simulink model "ImuCalibrator3Pass"  (R2018a)
settings: Solver=FixedStepDiscrete  StartTime=0.0  StopTime=inf  FixedStep=1/Fss  RelTol=1e-3
PreLoadFcn:
  | busDef
  | Fss = 1125;
  | Fss = 2100;
InitFcn:
  | modelDef = getModelDef(true);
undefined symbols (not defined in the file or in its folder): df, dw, Ggyr, Macc, Mgyr, numStates
libraries: simulink x15, vrlib x15, dspsigops x6, dspindex x6, dspinverses x6, dspstat3 x3, simulink_extras x3, dspmtrx3 x3, dspsrcs4 x3, dspmathops x3, dspswit3 x1
(part 1 of 4)
settings Model: Creator=Eric  LastModifiedBy=efoxlin
settings OptimizationCC: DefaultParameterBehavior=Inlined  InlineInvariantSignals=on  PassReuseOutputArgsAs=Individual arguments
settings DebuggingCC: ParameterTunabilityLossMsg=error  UnconnectedOutputMsg=none
settings SFSimCC: MATLABDynamicMemAlloc=off
settings RTWCC: SystemTargetFile=ert.tlc  TemplateMakefile=ert_default_tmf  GenerateReport=on  Toolchain=Microsoft Visual C++ 2017 v15.0 | nmake (64-bit Windows)  BuildConfiguration=Faster Runs  IncludeHyperlinkInReport=on  LaunchReport=on  GenerateTraceInfo=on  GenerateTraceReport=on  GenerateTraceReportSl=on  GenerateTraceReportSf=on  GenerateTraceReportEml=on
settings CodeAppCC: ForceParamTrailComments=on  IgnoreCustomStorageClasses=off  OperatorAnnotations=on  SimulinkDataObjDesc=on  SFDataObjDesc=on  InsertBlockDesc=on
settings ERTTargetCC: TargetLangStandard=C99 (ISO)  GenerateSampleERTMain=on  SupportComplex=off  SupportNonInlinedSFcns=on  SupportVariableSizeSignals=on  InlinedParameterPlacement=NonHierarchical  ERTCustomFileTemplate=example_file_process.tlc

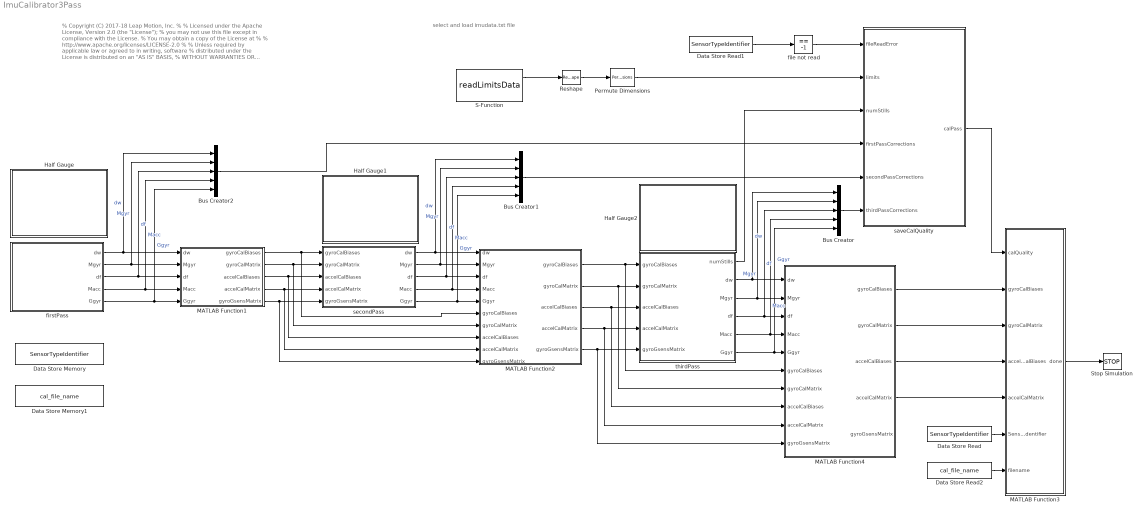
== system ImuCalibrator3Pass ==
  note: select and load imudata.txt file
  note: % Copyright (C) 2017-18 Leap Motion, Inc.
      | %
      | %    Licensed under the Apache License, Version 2.0 (the "License");
      | %    you may not use this file except in compliance with the License.
      | %    You may obtain a copy of the License at
      | %
      | %        http://www.apache.org/licenses/LICENSE-2.0
      | %
      | %    Unless required by applicable law or agreed to in writing, software
      | %    distributed under the License is distributed on an "AS IS" BASIS,
      | %    WITHOUT WARRANTIES OR CONDITIONS OF ANY KIND, either express or implied.
      | %    See the License for the specific language governing permissions and
      | %    limitations under the License.
      | % Author: Eric Foxlin
  Bus Creator : BusCreator  Inputs=dw,Mgyr,df,Macc,Ggyr
  Bus Creator1 : BusCreator  Inputs=dw,Mgyr,df,Macc,Ggyr
  Bus Creator2 : BusCreator  Inputs=dw,Mgyr,df,Macc,Ggyr
  Data Store Memory : DataStoreMemory  DataStoreName=SensorTypeIdentifier  ReadBeforeWriteMsg=warning  WriteAfterWriteMsg=warning  WriteAfterReadMsg=warning  InitialValue=-1  ShowAdditionalParam=off  OutDataTypeStr=int32
  Data Store Memory1 : DataStoreMemory  DataStoreName=cal_file_name  ReadBeforeWriteMsg=warning  WriteAfterWriteMsg=warning  WriteAfterReadMsg=warning  InitialValue=[76,69,48,48,48,48,48,48,48,48,48,48,48,48,48,48,48,48,45,48,48,48,48,45,48,48,48,48,48,48,48,48,48,48,45,105,109,117,46,106,115,111,110]  ShowAdditionalParam=off  OutDataTypeStr=uint8  Dimensions=[1,43]
  Data Store Read : DataStoreRead  Priority=7  DataStoreName=SensorTypeIdentifier
  Data Store Read1 : DataStoreRead  Priority=7  DataStoreName=SensorTypeIdentifier
  Data Store Read2 : DataStoreRead  Priority=7  DataStoreName=cal_file_name
  Half Gauge : Subsystem  DialogController=hmiCreateDDGDialog  IsWebBlock=on  mask(MWDashboardBlock){webBlockId=50db2cba-56c0-46f6-8461-fb1f4f79e19a, webBlockType=semicirculargauge, ShowInLibBrowser=on, ShowInitialText=on, HMISrcModelName=ImuCalibrator3Pass}
      mask prompts: webBlockId "WebBlock Id"; webBlockType "WebBlock Type"; HMISrcModelName "Source Model"
      mask help: SimulinkHMI:dialogs:SemicircularGaugeDialogDesc
      mask Help: helpview([docroot '/mapfiles/simulink.map'], 'hmi_half_gauge')
      mask Display:
      | if strcmp(get_param(bdroot(gcb),'BlockDiagramType'), 'library')
      |     image([(matlabroot) '/toolbox/simulink/hmi/icons/SemicircularGauge.png']);
      | end
  Half Gauge1 : Subsystem  DialogController=hmiCreateDDGDialog  IsWebBlock=on  mask(MWDashboardBlock){webBlockId=ea91a535-1150-4075-a79a-66e57a6dcc36, webBlockType=semicirculargauge, ShowInLibBrowser=on, ShowInitialText=on, HMISrcModelName=ImuCalibrator3Pass}
      mask prompts: webBlockId "WebBlock Id"; webBlockType "WebBlock Type"; HMISrcModelName "Source Model"
      mask help: SimulinkHMI:dialogs:SemicircularGaugeDialogDesc
      mask Help: helpview([docroot '/mapfiles/simulink.map'], 'hmi_half_gauge')
      mask Display:
      | if strcmp(get_param(bdroot(gcb),'BlockDiagramType'), 'library')
      |     image([(matlabroot) '/toolbox/simulink/hmi/icons/SemicircularGauge.png']);
      | end
  Half Gauge2 : Subsystem  DialogController=hmiCreateDDGDialog  IsWebBlock=on  mask(MWDashboardBlock){webBlockId=9f86d34f-810e-44c4-a7af-c4dea1104fb5, webBlockType=semicirculargauge, ShowInLibBrowser=on, ShowInitialText=on, HMISrcModelName=ImuCalibrator3Pass}
      mask prompts: webBlockId "WebBlock Id"; webBlockType "WebBlock Type"; HMISrcModelName "Source Model"
      mask help: SimulinkHMI:dialogs:SemicircularGaugeDialogDesc
      mask Help: helpview([docroot '/mapfiles/simulink.map'], 'hmi_half_gauge')
      mask Display:
      | if strcmp(get_param(bdroot(gcb),'BlockDiagramType'), 'library')
      |     image([(matlabroot) '/toolbox/simulink/hmi/icons/SemicircularGauge.png']);
      | end
  MATLAB Function1 : MATLAB Function  TreatAsAtomicUnit=on
  MATLAB Function2 : MATLAB Function  TreatAsAtomicUnit=on
  MATLAB Function3 : MATLAB Function  TreatAsAtomicUnit=on
  MATLAB Function4 : MATLAB Function  TreatAsAtomicUnit=on
  Permute Dimensions : PermuteDimensions
  Reshape : Reshape  OutputDimensionality=Customize  OutputDimensions=[6,3]
  S-Function : S-Function  FunctionName=readLimitsData  Parameters=-1  SFunctionDeploymentMode=off  EnableBusSupport=off
  Stop Simulation : Stop
  file not read : simulink/Logic and Bit Operations/Compare To Constant  relop===  const=-1  OutDataTypeStr=boolean
  firstPass : Subsystem  Priority=1
      mask init:
      | imuPar = getImuPar('lmvpUncalibrated');
  saveCalQuality : MATLAB Function  TreatAsAtomicUnit=on
  secondPass : Subsystem
      mask init:
      | imuPar = getImuPar('lmvp2ndPassCalibration');
  thirdPass : Subsystem
      mask init:
      | imuPar = getImuPar('lmvp2ndPassCalibration');
  wires:
  MATLAB Function1/1(gyroCalBiases) -> MATLAB Function2/6("gyroCalBiases "), secondPass/1(gyroCalBiases)
  MATLAB Function1/2(gyroCalMatrix) -> MATLAB Function2/7("gyroCalMatrix "), secondPass/2(gyroCalMatrix)
  MATLAB Function1/5(gyroGsensMatrix) -> MATLAB Function2/10("gyroGsensMatrix "), secondPass/5(gyroGsensMatrix)
  MATLAB Function1/3(accelCalBiases) -> MATLAB Function2/8("accelCalBiases "), secondPass/3(accelCalBiases)
  MATLAB Function1/4(accelCalMatrix) -> MATLAB Function2/9("accelCalMatrix "), secondPass/4(accelCalMatrix)
  MATLAB Function2/1(gyroCalBiases) -> MATLAB Function4/6("gyroCalBiases "), thirdPass/1(gyroCalBiases)
  MATLAB Function2/2(gyroCalMatrix) -> MATLAB Function4/7("gyroCalMatrix "), thirdPass/2(gyroCalMatrix)
  MATLAB Function2/3(accelCalBiases) -> MATLAB Function4/8("accelCalBiases "), thirdPass/3(accelCalBiases)
  MATLAB Function2/4(accelCalMatrix) -> MATLAB Function4/9("accelCalMatrix "), thirdPass/4(accelCalMatrix)
  MATLAB Function2/5(gyroGsensMatrix) -> MATLAB Function4/10("gyroGsensMatrix "), thirdPass/5(gyroGsensMatrix)
  thirdPass/2(dw) -> Bus Creator/1, MATLAB Function4/1(dw)  "dw"
  thirdPass/3(Mgyr) -> Bus Creator/2, MATLAB Function4/2(Mgyr)  "Mgyr"
  thirdPass/4(df) -> Bus Creator/3, MATLAB Function4/3(df)  "df"
  thirdPass/5(Macc) -> Bus Creator/4, MATLAB Function4/4(Macc)  "Macc"
  MATLAB Function4/1(gyroCalBiases) -> MATLAB Function3/2(gyroCalBiases)
  thirdPass/6(Ggyr) -> Bus Creator/5, MATLAB Function4/5(Ggyr)  "Ggyr"
  MATLAB Function3/1(done) -> Stop Simulation/1
  Bus Creator/1 -> saveCalQuality/6(thirdPassCorrections)
  MATLAB Function4/2(gyroCalMatrix) -> MATLAB Function3/3(gyroCalMatrix)
  MATLAB Function4/3(accelCalBiases) -> MATLAB Function3/4(accelCalBiases)
  MATLAB Function4/4(accelCalMatrix) -> MATLAB Function3/5(accelCalMatrix)
  saveCalQuality/1(calPass) -> MATLAB Function3/1(calQuality)
  secondPass/5(Ggyr) -> Bus Creator1/5, MATLAB Function2/5(Ggyr)  "Ggyr"
  secondPass/3(df) -> Bus Creator1/3, MATLAB Function2/3(df)  "df"
  secondPass/4(Macc) -> Bus Creator1/4, MATLAB Function2/4(Macc)  "Macc"
  secondPass/2(Mgyr) -> Bus Creator1/2, MATLAB Function2/2(Mgyr)  "Mgyr"
  secondPass/1(dw) -> Bus Creator1/1, MATLAB Function2/1(dw)  "dw"
  firstPass/1(dw) -> Bus Creator2/1, MATLAB Function1/1(dw)  "dw"
  firstPass/2(Mgyr) -> Bus Creator2/2, MATLAB Function1/2(Mgyr)  "Mgyr"
  firstPass/4(Macc) -> Bus Creator2/4, MATLAB Function1/4(Macc)  "Macc"
  firstPass/3(df) -> Bus Creator2/3, MATLAB Function1/3(df)  "df"
  firstPass/5(Ggyr) -> Bus Creator2/5, MATLAB Function1/5(Ggyr)  "Ggyr"
  Bus Creator1/1 -> saveCalQuality/5(secondPassCorrections)
  Bus Creator2/1 -> saveCalQuality/4(firstPassCorrections)
  Data Store Read/1 -> MATLAB Function3/6(SensorTypeIdentifier)
  Data Store Read1/1 -> file not read/1
  file not read/1 -> saveCalQuality/1(fileReadError)
  thirdPass/1(numStills) -> saveCalQuality/3(numStills)
  Permute Dimensions/1 -> saveCalQuality/2(limits)
  S-Function/1 -> Reshape/1
  Reshape/1 -> Permute Dimensions/1
  Data Store Read2/1 -> MATLAB Function3/7(filename)

== system ImuCalibrator3Pass/Half Gauge ==

== system ImuCalibrator3Pass/Half Gauge1 ==

== system ImuCalibrator3Pass/Half Gauge2 ==

== system ImuCalibrator3Pass/firstPass ==
  AINS : Subsystem  TreatAsAtomicUnit=on
  Binary File Reader : dspsrcs4/Binary File Reader  Commented=on  Filename=GyroAccelDtFloat32.bin  HeaderStructure=struct([])  DataType=single  SamplesPerFrame=1  IsDataComplex=off  NumChannels=7  OutputEOF=on  SampleTime=-1  SimulateUsing=Code generation
      settings: SourceProductName=DSP System Toolbox  SourceProductBaseCode=DS
  Bus Selector : BusSelector  OutputSignals=dw,Mgyr,df,Macc,Ggyr
  Compare To Zero : simulink/Logic and Bit Operations/Compare To Zero  relop===  OutDataTypeStr=boolean
  Constant : Constant  Value=int32(4096)
  Cumulative time : dspmathops/Cumulative Sum  dim=Channels (running sum)  reset_popup=None  roundingMode=Floor  overflowMode=off  outputDataTypeStr=Inherit: Same as accumulator  outputMin=[]  outputMax=[]  outputLastDataTypeStr=Inherit: Same as accumulator
      settings: SourceProductName=DSP System Toolbox
  Data Type Conversion : DataTypeConversion
  Demux : Demux  Outputs=[3 3 1]
  Dt : Selector  InputPortWidth=7  IndexOptions=Index vector (dialog)  Indices=7  OutputSizes=1
  Logical Operator : Logic  Operator=NOT  AllPortsSameDT=off  OutDataTypeStr=boolean
  MATLAB Function1 : MATLAB Function  Commented=on  TreatAsAtomicUnit=on
  Math Function : Math  Operator=mod  SaturateOnIntegerOverflow=on
  Reshape : Reshape  OutputDimensionality=Column vector (2-D)
  Scope1 : Scope
  Scope10 : Scope
  Scope3 : Scope
  To Workspace : ToWorkspace  Commented=on  VariableName=simout  SaveFormat=Timeseries  SampleTime=-1
      settings: Save2DSignal=2-D array (concatenate along first dimension)
  While Iterator : WhileIterator  MaxIters=500000  WhileBlockType=do-while  ShowIterationPort=on
  printTime : Subsystem
  readImuData : Subsystem
  dw : Outport
  Mgyr : Outport  Port=2
  df : Outport  Port=3
  Macc : Outport  Port=4
  Ggyr : Outport  Port=5
  wires:
  AINS/1(filterOut) -> Bus Selector/1, To Workspace/1  "filterOut"
  Demux/1 -> AINS/1(w_ib^b), Scope1/1
  Demux/3 -> Scope3/1, AINS/3(Dt)
  Demux/2 -> AINS/2(f_ib^b), Scope10/1
  Bus Selector/1 -> dw/1  "<dw>"
  Bus Selector/2 -> Mgyr/1  "<Mgyr>"
  Bus Selector/3 -> df/1  "<df>"
  Bus Selector/4 -> Macc/1  "<Macc>"
  Bus Selector/5 -> Ggyr/1  "<Ggyr>"
  While Iterator/1 -> Math Function/1
  Math Function/1 -> Compare To Zero/1
  Constant/1 -> Math Function/2
  Cumulative time/1 -> printTime/1(time)  "firstPassTime"
  readImuData/1(GyrosAccelsDt) -> Data Type Conversion/1
  Reshape/1 -> Demux/1
  readImuData/2(EOF) -> Logical Operator/1
  Logical Operator/1 -> While Iterator/1
  Data Type Conversion/1 -> Dt/1, Reshape/1
  Compare To Zero/1 -> printTime/Enable
  Dt/1 -> Cumulative time/1

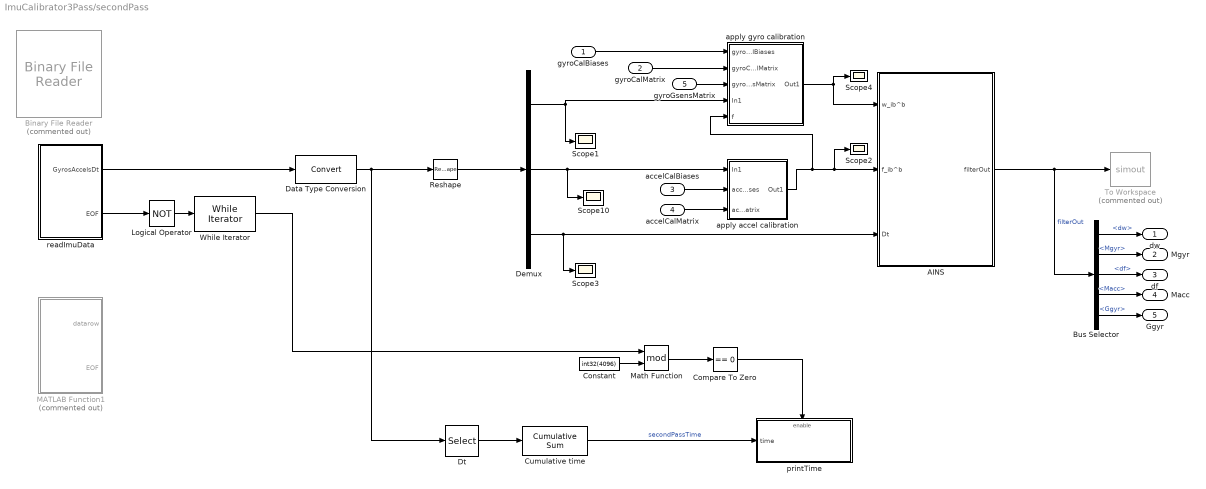
== system ImuCalibrator3Pass/secondPass ==
  gyroCalBiases : Inport
  gyroCalMatrix : Inport  Port=2
  accelCalBiases : Inport  Port=3
  accelCalMatrix : Inport  Port=4
  gyroGsensMatrix : Inport  Port=5
  AINS : Subsystem  TreatAsAtomicUnit=on
  Binary File Reader : dspsrcs4/Binary File Reader  Commented=on  Filename=GyroAccelDtFloat32.bin  HeaderStructure=struct([])  DataType=single  SamplesPerFrame=1  IsDataComplex=off  NumChannels=7  OutputEOF=on  SampleTime=-1  SimulateUsing=Code generation
      settings: SourceProductName=DSP System Toolbox  SourceProductBaseCode=DS
  Bus Selector : BusSelector  OutputSignals=dw,Mgyr,df,Macc,Ggyr
  Compare To Zero : simulink/Logic and Bit Operations/Compare To Zero  relop===  OutDataTypeStr=boolean
  Constant : Constant  Value=int32(4096)
  Cumulative time : dspmathops/Cumulative Sum  dim=Channels (running sum)  reset_popup=None  roundingMode=Floor  overflowMode=off  outputDataTypeStr=Inherit: Same as accumulator  outputMin=[]  outputMax=[]  outputLastDataTypeStr=Inherit: Same as accumulator
      settings: SourceProductName=DSP System Toolbox
  Data Type Conversion : DataTypeConversion
  Demux : Demux  Outputs=[3 3 1]
  Dt : Selector  InputPortWidth=7  IndexOptions=Index vector (dialog)  Indices=7  OutputSizes=1
  Logical Operator : Logic  Operator=NOT  AllPortsSameDT=off  OutDataTypeStr=boolean
  MATLAB Function1 : MATLAB Function  Commented=on  TreatAsAtomicUnit=on
  Math Function : Math  Operator=mod  SaturateOnIntegerOverflow=on
  Reshape : Reshape  OutputDimensionality=Column vector (2-D)
  Scope{1..4,10} (5 alike) : Scope
  To Workspace : ToWorkspace  Commented=on  VariableName=simout  SaveFormat=Timeseries  SampleTime=-1
      settings: Save2DSignal=2-D array (concatenate along first dimension)
  While Iterator : WhileIterator  MaxIters=500000  WhileBlockType=do-while  ShowIterationPort=on
  apply accel calibration : Subsystem  TreatAsAtomicUnit=on
  apply gyro calibration : Subsystem  TreatAsAtomicUnit=on
  printTime : Subsystem
  readImuData : Subsystem
  dw : Outport
  Mgyr : Outport  Port=2
  df : Outport  Port=3
  Macc : Outport  Port=4
  Ggyr : Outport  Port=5
  wires:
  Compare To Zero/1 -> printTime/Enable
  Data Type Conversion/1 -> Dt/1, Reshape/1
  Logical Operator/1 -> While Iterator/1
  readImuData/2(EOF) -> Logical Operator/1
  Reshape/1 -> Demux/1
  readImuData/1(GyrosAccelsDt) -> Data Type Conversion/1
  Cumulative time/1 -> printTime/1(time)  "secondPassTime"
  Constant/1 -> Math Function/2
  Math Function/1 -> Compare To Zero/1
  While Iterator/1 -> Math Function/1
  Bus Selector/5 -> Ggyr/1  "<Ggyr>"
  Bus Selector/4 -> Macc/1  "<Macc>"
  Bus Selector/3 -> df/1  "<df>"
  Bus Selector/2 -> Mgyr/1  "<Mgyr>"
  Bus Selector/1 -> dw/1  "<dw>"
  apply accel calibration/1(Out1) -> apply gyro calibration/5(f), Scope2/1, AINS/2(f_ib^b)
  Demux/3 -> AINS/3(Dt), Scope3/1
  apply gyro calibration/1(Out1) -> AINS/1(w_ib^b), Scope4/1
  Demux/1 -> apply gyro calibration/4(In1), Scope1/1
  Demux/2 -> apply accel calibration/1(In1), Scope10/1
  AINS/1(filterOut) -> To Workspace/1, Bus Selector/1  "filterOut"
  gyroCalBiases/1 -> apply gyro calibration/1(gyroCalBiases)
  gyroCalMatrix/1 -> apply gyro calibration/2(gyroCalMatrix)
  gyroGsensMatrix/1 -> apply gyro calibration/3(gyroGsensMatrix)
  accelCalBiases/1 -> apply accel calibration/2(accelCalBiases)
  accelCalMatrix/1 -> apply accel calibration/3(accelCalMatrix)
  Dt/1 -> Cumulative time/1

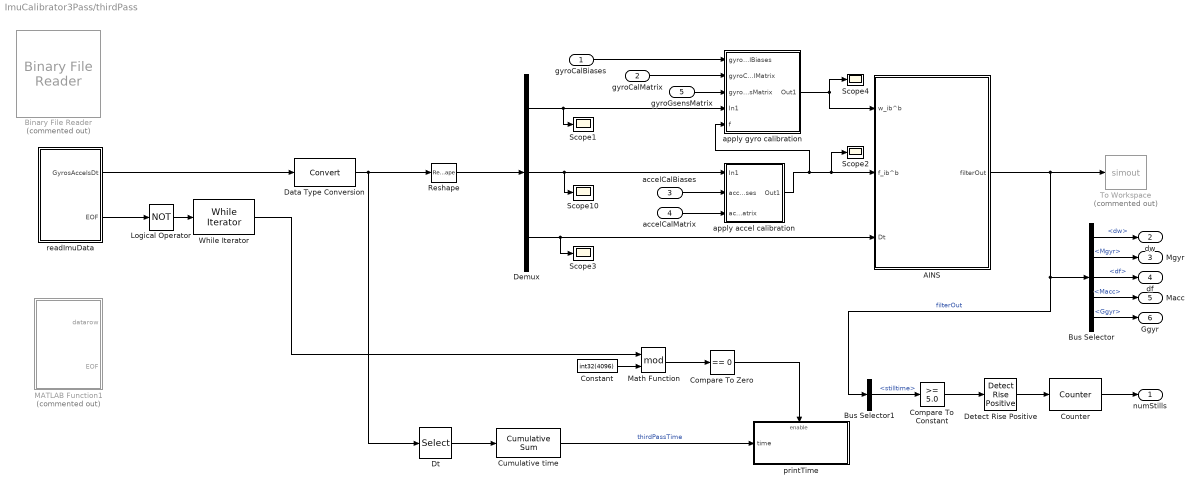
== system ImuCalibrator3Pass/thirdPass ==
  gyroCalBiases : Inport
  gyroCalMatrix : Inport  Port=2
  accelCalBiases : Inport  Port=3
  accelCalMatrix : Inport  Port=4
  gyroGsensMatrix : Inport  Port=5
  AINS : Subsystem  TreatAsAtomicUnit=on
  Binary File Reader : dspsrcs4/Binary File Reader  Commented=on  Filename=GyroAccelDtFloat32.bin  HeaderStructure=struct([])  DataType=single  SamplesPerFrame=1  IsDataComplex=off  NumChannels=7  OutputEOF=on  SampleTime=-1  SimulateUsing=Code generation
      settings: SourceProductName=DSP System Toolbox  SourceProductBaseCode=DS
  Bus Selector : BusSelector  OutputSignals=dw,Mgyr,df,Macc,Ggyr
  Bus Selector1 : BusSelector  OutputSignals=stilltime
  Compare To Constant : simulink/Logic and Bit Operations/Compare To Constant  relop=>=  const=5.0  OutDataTypeStr=boolean
  Compare To Zero : simulink/Logic and Bit Operations/Compare To Zero  relop===  OutDataTypeStr=boolean
  Constant : Constant  Value=int32(4096)
  Counter : dspswit3/Counter  Direction=Up  CountEvent=Non-zero sample  CounterSize=User defined  MaxCount=255  InitialCount=0  Output=Count  HitValue=32  ResetInput=off  SamplesPerFrame=1  Ts=1  CntDtype=double  HitDtype=Logical
  Cumulative time : dspmathops/Cumulative Sum  dim=Channels (running sum)  reset_popup=None  roundingMode=Floor  overflowMode=off  outputDataTypeStr=Inherit: Same as accumulator  outputMin=[]  outputMax=[]  outputLastDataTypeStr=Inherit: Same as accumulator
      settings: SourceProductName=DSP System Toolbox
  Data Type Conversion : DataTypeConversion
  Demux : Demux  Outputs=[3 3 1]
  Detect Rise Positive : simulink/Logic and Bit Operations/Detect Rise Positive  vinit=0  OutDataTypeStr=boolean
  Dt : Selector  InputPortWidth=7  IndexOptions=Index vector (dialog)  Indices=7  OutputSizes=1
  Logical Operator : Logic  Operator=NOT  AllPortsSameDT=off  OutDataTypeStr=boolean
  MATLAB Function1 : MATLAB Function  Commented=on  TreatAsAtomicUnit=on
  Math Function : Math  Operator=mod  SaturateOnIntegerOverflow=on
  Reshape : Reshape  OutputDimensionality=Column vector (2-D)
  Scope{1..4,10} (5 alike) : Scope
  To Workspace : ToWorkspace  Commented=on  VariableName=simout  SaveFormat=Timeseries  SampleTime=-1
      settings: Save2DSignal=2-D array (concatenate along first dimension)
  While Iterator : WhileIterator  MaxIters=500000  WhileBlockType=do-while  ShowIterationPort=on
  apply accel calibration : Subsystem  TreatAsAtomicUnit=on
  apply gyro calibration : Subsystem  TreatAsAtomicUnit=on
  printTime : Subsystem
  readImuData : Subsystem
  numStills : Outport  InitialOutput=0
  dw : Outport  Port=2
  Mgyr : Outport  Port=3
  df : Outport  Port=4
  Macc : Outport  Port=5
  Ggyr : Outport  Port=6
  wires:
  accelCalMatrix/1 -> apply accel calibration/3(accelCalMatrix)
  accelCalBiases/1 -> apply accel calibration/2(accelCalBiases)
  gyroGsensMatrix/1 -> apply gyro calibration/3(gyroGsensMatrix)
  gyroCalMatrix/1 -> apply gyro calibration/2(gyroCalMatrix)
  gyroCalBiases/1 -> apply gyro calibration/1(gyroCalBiases)
  AINS/1(filterOut) -> Bus Selector1/1, Bus Selector/1, To Workspace/1  "filterOut"
  Demux/2 -> Scope10/1, apply accel calibration/1(In1)
  Demux/1 -> Scope1/1, apply gyro calibration/4(In1)
  apply gyro calibration/1(Out1) -> Scope4/1, AINS/1(w_ib^b)
  Demux/3 -> Scope3/1, AINS/3(Dt)
  apply accel calibration/1(Out1) -> AINS/2(f_ib^b), Scope2/1, apply gyro calibration/5(f)
  Bus Selector/1 -> dw/1  "<dw>"
  Bus Selector/2 -> Mgyr/1  "<Mgyr>"
  Bus Selector/3 -> df/1  "<df>"
  Bus Selector/4 -> Macc/1  "<Macc>"
  Bus Selector/5 -> Ggyr/1  "<Ggyr>"
  While Iterator/1 -> Math Function/1
  Math Function/1 -> Compare To Zero/1
  Constant/1 -> Math Function/2
  Cumulative time/1 -> printTime/1(time)  "thirdPassTime"
  readImuData/1(GyrosAccelsDt) -> Data Type Conversion/1
  Reshape/1 -> Demux/1
  readImuData/2(EOF) -> Logical Operator/1
  Logical Operator/1 -> While Iterator/1
  Data Type Conversion/1 -> Dt/1, Reshape/1
  Compare To Zero/1 -> printTime/Enable
  Dt/1 -> Cumulative time/1
  Bus Selector1/1 -> Compare To Constant/1  "<stilltime>"
  Compare To Constant/1 -> Detect Rise Positive/1
  Detect Rise Positive/1 -> Counter/1
  Counter/1 -> numStills/1

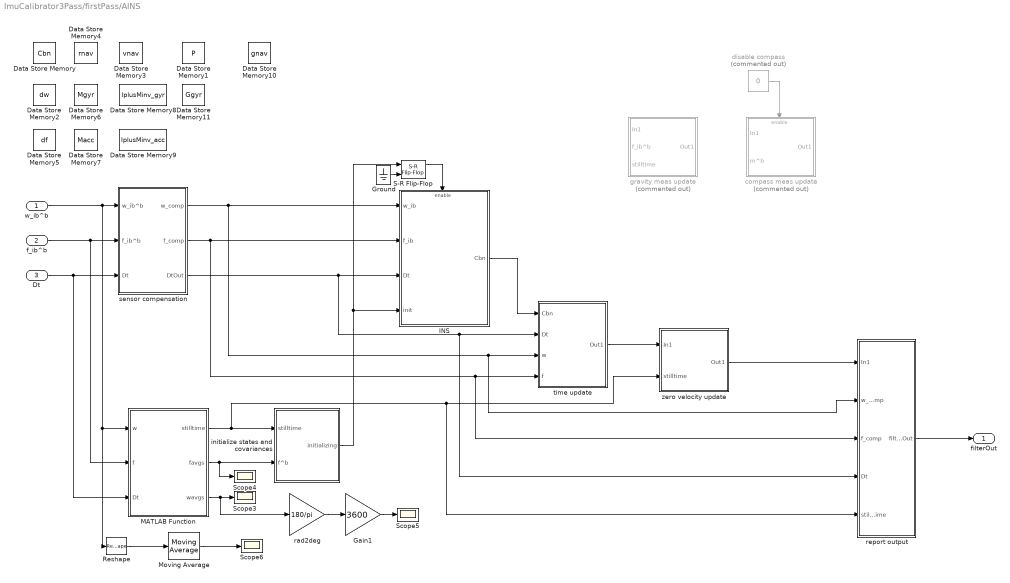
== system ImuCalibrator3Pass/firstPass/AINS ==
  w_ib^b : Inport  Unit=rad/s
  f_ib^b : Inport  Port=2  Unit=m/s^2  PortDimensions=3
  Dt : Inport  Port=3  Unit=rad/s
  Data Store Memory : DataStoreMemory  DataStoreName=Cbn  ReadBeforeWriteMsg=warning  WriteAfterWriteMsg=warning  WriteAfterReadMsg=warning  InitialValue=eye(3)  VectorParams1D=off  ShowAdditionalParam=off
  Data Store Memory1 : DataStoreMemory  DataStoreName=P  ReadBeforeWriteMsg=warning  WriteAfterWriteMsg=warning  WriteAfterReadMsg=warning  InitialValue=eye(modelDef.numStates)*1e-12  ShowAdditionalParam=off
  Data Store Memory10 : DataStoreMemory  DataStoreName=gnav  ReadBeforeWriteMsg=warning  WriteAfterWriteMsg=warning  WriteAfterReadMsg=warning  InitialValue=[0;0; 9.8065]  VectorParams1D=off  ShowAdditionalParam=off
  Data Store Memory11 : DataStoreMemory  DataStoreName=Ggyr  ReadBeforeWriteMsg=warning  WriteAfterWriteMsg=warning  WriteAfterReadMsg=warning  InitialValue=zeros(3,3)  VectorParams1D=off  ShowAdditionalParam=off
  Data Store Memory2 : DataStoreMemory  DataStoreName=dw  ReadBeforeWriteMsg=warning  WriteAfterWriteMsg=warning  WriteAfterReadMsg=warning  InitialValue=[0;0;0]  VectorParams1D=off  ShowAdditionalParam=off
  Data Store Memory3 : DataStoreMemory  DataStoreName=vnav  ReadBeforeWriteMsg=warning  WriteAfterWriteMsg=warning  WriteAfterReadMsg=warning  InitialValue=[0;0;0]  VectorParams1D=off  ShowAdditionalParam=off
  Data Store Memory4 : DataStoreMemory  DataStoreName=rnav  ReadBeforeWriteMsg=warning  WriteAfterWriteMsg=warning  WriteAfterReadMsg=warning  InitialValue=[0;0;0]  VectorParams1D=off  ShowAdditionalParam=off
  Data Store Memory5 : DataStoreMemory  DataStoreName=df  ReadBeforeWriteMsg=warning  WriteAfterWriteMsg=warning  WriteAfterReadMsg=warning  InitialValue=[0;0;0]  VectorParams1D=off  ShowAdditionalParam=off
  Data Store Memory6 : DataStoreMemory  DataStoreName=Mgyr  ReadBeforeWriteMsg=warning  WriteAfterWriteMsg=warning  WriteAfterReadMsg=warning  InitialValue=zeros(3,3)  VectorParams1D=off  ShowAdditionalParam=off
  Data Store Memory7 : DataStoreMemory  DataStoreName=Macc  ReadBeforeWriteMsg=warning  WriteAfterWriteMsg=warning  WriteAfterReadMsg=warning  InitialValue=zeros(3,3)  VectorParams1D=off  ShowAdditionalParam=off
  Data Store Memory8 : DataStoreMemory  DataStoreName=IplusMinv_gyr  ReadBeforeWriteMsg=warning  WriteAfterWriteMsg=warning  WriteAfterReadMsg=warning  InitialValue=eye(3)  VectorParams1D=off  ShowAdditionalParam=off
  Data Store Memory9 : DataStoreMemory  DataStoreName=IplusMinv_acc  ReadBeforeWriteMsg=warning  WriteAfterWriteMsg=warning  WriteAfterReadMsg=warning  InitialValue=eye(3)  VectorParams1D=off  ShowAdditionalParam=off
  Gain1 : Gain  Gain=3600
  Ground : Ground
  INS : Subsystem  Priority=2
  MATLAB Function : MATLAB Function  TreatAsAtomicUnit=on
  Moving Average : dspstat3/Moving Average  Method=Sliding window  ForgettingFactorPort=off  SpecifyWindowLength=on  WindowLength=1000  ForgettingFactor=0.9  SimulateUsing=Code generation
  Reshape : Reshape  OutputDimensionality=Row vector (2-D)
  S-R Flip-Flop : simulink_extras/Flip Flops/S-R Flip-Flop  initial_condition=0
  Scope{3..6} (4 alike) : Scope
  compass meas update : Subsystem  Commented=on  TreatAsAtomicUnit=on
  disable compass : Constant  Commented=on  Value=0
  gravity meas update : Subsystem  Commented=on  TreatAsAtomicUnit=on
  initialize states and covariances : Subsystem  Priority=1  TreatAsAtomicUnit=on
  rad2deg : Gain  Gain=180/pi
  report output : Subsystem  Priority=10  TreatAsAtomicUnit=on
  sensor compensation : Subsystem
  time update : Subsystem  Priority=3  TreatAsAtomicUnit=on
  zero velocity update : Subsystem  Priority=4  TreatAsAtomicUnit=on
  filterOut : Outport
  wires:
  time update/1(Out1) -> zero velocity update/1(In1)
  disable compass/1 -> compass meas update/Enable
  MATLAB Function/1(stilltime) -> report output/5(stilltime), zero velocity update/2(stilltime), initialize states and covariances/1(stilltime)
  MATLAB Function/2(favgs) -> Scope4/1, initialize states and covariances/2(f^b)
  zero velocity update/1(Out1) -> report output/1(In1)
  sensor compensation/1(w_comp) -> report output/2(w_comp), time update/3(w), INS/1(w_ib)
  INS/1(Cbn) -> time update/1(Cbn)
  sensor compensation/3(DtOut) -> report output/4(Dt), time update/2(Dt), INS/3(Dt)
  sensor compensation/2(f_comp) -> INS/2(f_ib), report output/3(f_comp), time update/4(f)
  f_ib^b/1 -> MATLAB Function/2(f), sensor compensation/2(f_ib^b)
  w_ib^b/1 -> MATLAB Function/1(w), Reshape/1, sensor compensation/1(w_ib^b)
  Dt/1 -> MATLAB Function/3(Dt), sensor compensation/3(Dt)
  initialize states and covariances/1(initializing) -> INS/4(init), S-R Flip-Flop/1
  MATLAB Function/3(wavgs) -> rad2deg/1, Scope3/1
  rad2deg/1 -> Gain1/1
  Gain1/1 -> Scope5/1
  Moving Average/1 -> Scope6/1
  Reshape/1 -> Moving Average/1
  S-R Flip-Flop/1 -> INS/Enable
  report output/1(filterOut) -> filterOut/1
  Ground/1 -> S-R Flip-Flop/2

== system ImuCalibrator3Pass/firstPass/printTime ==
  time : Inport
  Enable : EnablePort
  MATLAB Function : MATLAB Function  TreatAsAtomicUnit=on
  wires:
  time/1 -> MATLAB Function/1(u)

== system ImuCalibrator3Pass/firstPass/readImuData ==
  C++ S-function : S-Function  FunctionName=readImuData  Parameters=-1  SFunctionDeploymentMode=off  EnableBusSupport=off
  Constant : Constant  Value=0
  Constant1 : Constant
  Data Store Read : DataStoreRead  DataStoreName=SensorTypeIdentifier
  Data Store Write : DataStoreWrite  DataStoreName=cal_file_name
  Data Type Conversion : DataTypeConversion
  Data Type Conversion1 : DataTypeConversion  OutDataTypeStr=uint8
  Difference1 : simulink/Discrete/Difference  ICPrevInput=0.0  OutMin=[]  OutMax=[]  OutDataType=fixdt(1, 16)  OutScaling=2^-10  DoSatur=off
  Mux : Mux  Inputs=2
  SensorType : Selector  InputPortWidth=11  IndexOptions=Index vector (dialog)  Indices=2  OutputSizes=1
  Unit Delay : UnitDelay  SampleTime=-1
  Unit Delay1 : UnitDelay  SampleTime=-1
  avoid huge jump on first cycle : Switch  Criteria=u2 > Threshold  Threshold=0.5
  avoid sending garbage on the last row : Switch  Criteria=u2 > Threshold  Threshold=0.5
  gyros accels : Selector  InputPortWidth=11  IndexOptions=Index vector (dialog)  Indices=[5:10]  OutputSizes=1
  not initialized : simulink/Logic and Bit Operations/Compare To Constant  relop===  const=-1  OutDataTypeStr=boolean
  tstamp : Selector  InputPortWidth=11  IndexOptions=Index vector (dialog)  Indices=3  OutputSizes=1
  write SensorTypeIdentifier once : Subsystem  TreatAsAtomicUnit=on
  GyrosAccelsDt : Outport
  EOF : Outport  Port=2
  wires:
  tstamp/1 -> Difference1/1
  C++ S-function/1 -> gyros accels/1, SensorType/1, tstamp/1
  gyros accels/1 -> Mux/1
  SensorType/1 -> Data Type Conversion/1
  Data Store Read/1 -> not initialized/1
  not initialized/1 -> write SensorTypeIdentifier once/Enable
  Data Type Conversion/1 -> write SensorTypeIdentifier once/1(In1)
  Unit Delay/1 -> avoid sending garbage on the last row/1
  C++ S-function/2 -> avoid sending garbage on the last row/2, EOF/1
  avoid sending garbage on the last row/1 -> GyrosAccelsDt/1
  Mux/1 -> Unit Delay/1, avoid sending garbage on the last row/3
  Unit Delay1/1 -> avoid huge jump on first cycle/2
  Difference1/1 -> avoid huge jump on first cycle/1
  Constant/1 -> avoid huge jump on first cycle/3
  Constant1/1 -> Unit Delay1/1
  avoid huge jump on first cycle/1 -> Mux/2
  ? -> Data Type Conversion1/1
  Data Type Conversion1/1 -> Data Store Write/1

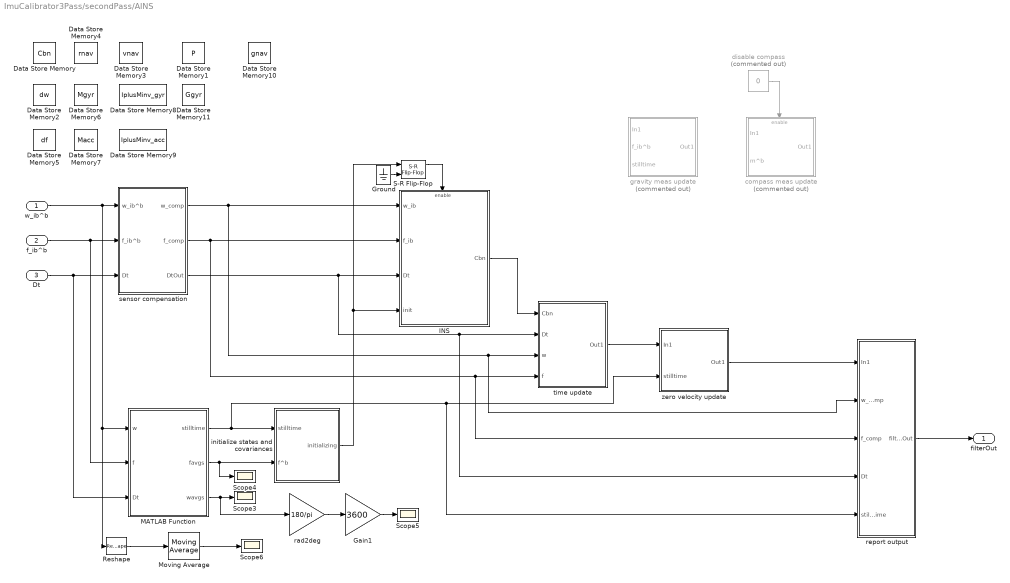
== system ImuCalibrator3Pass/secondPass/AINS ==
  w_ib^b : Inport  Unit=rad/s
  f_ib^b : Inport  Port=2  Unit=m/s^2  PortDimensions=3
  Dt : Inport  Port=3  Unit=rad/s
  Data Store Memory : DataStoreMemory  DataStoreName=Cbn  ReadBeforeWriteMsg=warning  WriteAfterWriteMsg=warning  WriteAfterReadMsg=warning  InitialValue=eye(3)  VectorParams1D=off  ShowAdditionalParam=off
  Data Store Memory1 : DataStoreMemory  DataStoreName=P  ReadBeforeWriteMsg=warning  WriteAfterWriteMsg=warning  WriteAfterReadMsg=warning  InitialValue=eye(modelDef.numStates)*1e-12  ShowAdditionalParam=off
  Data Store Memory10 : DataStoreMemory  DataStoreName=gnav  ReadBeforeWriteMsg=warning  WriteAfterWriteMsg=warning  WriteAfterReadMsg=warning  InitialValue=[0;0; 9.8065]  VectorParams1D=off  ShowAdditionalParam=off
  Data Store Memory11 : DataStoreMemory  DataStoreName=Ggyr  ReadBeforeWriteMsg=warning  WriteAfterWriteMsg=warning  WriteAfterReadMsg=warning  InitialValue=zeros(3,3)  VectorParams1D=off  ShowAdditionalParam=off
  Data Store Memory2 : DataStoreMemory  DataStoreName=dw  ReadBeforeWriteMsg=warning  WriteAfterWriteMsg=warning  WriteAfterReadMsg=warning  InitialValue=[0;0;0]  VectorParams1D=off  ShowAdditionalParam=off
  Data Store Memory3 : DataStoreMemory  DataStoreName=vnav  ReadBeforeWriteMsg=warning  WriteAfterWriteMsg=warning  WriteAfterReadMsg=warning  InitialValue=[0;0;0]  VectorParams1D=off  ShowAdditionalParam=off
  Data Store Memory4 : DataStoreMemory  DataStoreName=rnav  ReadBeforeWriteMsg=warning  WriteAfterWriteMsg=warning  WriteAfterReadMsg=warning  InitialValue=[0;0;0]  VectorParams1D=off  ShowAdditionalParam=off
  Data Store Memory5 : DataStoreMemory  DataStoreName=df  ReadBeforeWriteMsg=warning  WriteAfterWriteMsg=warning  WriteAfterReadMsg=warning  InitialValue=[0;0;0]  VectorParams1D=off  ShowAdditionalParam=off
  Data Store Memory6 : DataStoreMemory  DataStoreName=Mgyr  ReadBeforeWriteMsg=warning  WriteAfterWriteMsg=warning  WriteAfterReadMsg=warning  InitialValue=zeros(3,3)  VectorParams1D=off  ShowAdditionalParam=off
  Data Store Memory7 : DataStoreMemory  DataStoreName=Macc  ReadBeforeWriteMsg=warning  WriteAfterWriteMsg=warning  WriteAfterReadMsg=warning  InitialValue=zeros(3,3)  VectorParams1D=off  ShowAdditionalParam=off
  Data Store Memory8 : DataStoreMemory  DataStoreName=IplusMinv_gyr  ReadBeforeWriteMsg=warning  WriteAfterWriteMsg=warning  WriteAfterReadMsg=warning  InitialValue=eye(3)  VectorParams1D=off  ShowAdditionalParam=off
  Data Store Memory9 : DataStoreMemory  DataStoreName=IplusMinv_acc  ReadBeforeWriteMsg=warning  WriteAfterWriteMsg=warning  WriteAfterReadMsg=warning  InitialValue=eye(3)  VectorParams1D=off  ShowAdditionalParam=off
  Gain1 : Gain  Gain=3600
  Ground : Ground
  INS : Subsystem  Priority=2
  MATLAB Function : MATLAB Function  TreatAsAtomicUnit=on
  Moving Average : dspstat3/Moving Average  Method=Sliding window  ForgettingFactorPort=off  SpecifyWindowLength=on  WindowLength=1000  ForgettingFactor=0.9  SimulateUsing=Code generation
  Reshape : Reshape  OutputDimensionality=Row vector (2-D)
  S-R Flip-Flop : simulink_extras/Flip Flops/S-R Flip-Flop  initial_condition=0
  Scope{3..6} (4 alike) : Scope
  compass meas update : Subsystem  Commented=on  TreatAsAtomicUnit=on
  disable compass : Constant  Commented=on  Value=0
  gravity meas update : Subsystem  Commented=on  TreatAsAtomicUnit=on
  initialize states and covariances : Subsystem  Priority=1  TreatAsAtomicUnit=on
  rad2deg : Gain  Gain=180/pi
  report output : Subsystem  Priority=10  TreatAsAtomicUnit=on
  sensor compensation : Subsystem
  time update : Subsystem  Priority=3  TreatAsAtomicUnit=on
  zero velocity update : Subsystem  Priority=4  TreatAsAtomicUnit=on
  filterOut : Outport
  wires:
  Ground/1 -> S-R Flip-Flop/2
  report output/1(filterOut) -> filterOut/1
  S-R Flip-Flop/1 -> INS/Enable
  Reshape/1 -> Moving Average/1
  Moving Average/1 -> Scope6/1
  Gain1/1 -> Scope5/1
  rad2deg/1 -> Gain1/1
  MATLAB Function/3(wavgs) -> Scope3/1, rad2deg/1
  initialize states and covariances/1(initializing) -> S-R Flip-Flop/1, INS/4(init)
  Dt/1 -> sensor compensation/3(Dt), MATLAB Function/3(Dt)
  w_ib^b/1 -> sensor compensation/1(w_ib^b), Reshape/1, MATLAB Function/1(w)
  f_ib^b/1 -> sensor compensation/2(f_ib^b), MATLAB Function/2(f)
  sensor compensation/2(f_comp) -> time update/4(f), report output/3(f_comp), INS/2(f_ib)
  sensor compensation/3(DtOut) -> INS/3(Dt), time update/2(Dt), report output/4(Dt)
  INS/1(Cbn) -> time update/1(Cbn)
  sensor compensation/1(w_comp) -> INS/1(w_ib), time update/3(w), report output/2(w_comp)
  zero velocity update/1(Out1) -> report output/1(In1)
  MATLAB Function/2(favgs) -> initialize states and covariances/2(f^b), Scope4/1
  MATLAB Function/1(stilltime) -> initialize states and covariances/1(stilltime), zero velocity update/2(stilltime), report output/5(stilltime)
  disable compass/1 -> compass meas update/Enable
  time update/1(Out1) -> zero velocity update/1(In1)

== system ImuCalibrator3Pass/secondPass/apply accel calibration ==
  In1 : Inport
  accelCalBiases : Inport  Port=2
  accelCalMatrix : Inport  Port=3
  "Accel SFMA matrix, column-major1" : Constant  Value="[0.9973\t0.0126\t0.0025\t0.0004\t1.0177\t0.003\t0.0064\t0.0308\t1.0224]"  VectorParams1D=off
  Matrix Multiply : Product  Multiplication=Matrix(*)
  Sum : Sum  Inputs=|+-
  Out1 : Outport
  wires:
  accelCalMatrix/1 -> Matrix Multiply/1
  accelCalBiases/1 -> Sum/2
  Sum/1 -> Matrix Multiply/2
  Matrix Multiply/1 -> Out1/1
  In1/1 -> Sum/1

== system ImuCalibrator3Pass/secondPass/apply gyro calibration ==
  gyroCalBiases : Inport
  gyroCalMatrix : Inport  Port=2
  gyroGsensMatrix : Inport  Port=3
  In1 : Inport  Port=4
  f : Inport  Port=5
  "Accel SFMA matrix, column-major1" : Constant  Value="[0.9973\t0.0126\t0.0025\t0.0004\t1.0177\t0.003\t0.0064\t0.0308\t1.0224]"  VectorParams1D=off
  Matrix Multiply : Product  Multiplication=Matrix(*)
  Matrix Multiply1 : Product  Multiplication=Matrix(*)
  Sum : Sum  Inputs=|+-
  Sum1 : Sum  Inputs=|+-
  Out1 : Outport
  wires:
  gyroGsensMatrix/1 -> Matrix Multiply1/1
  f/1 -> Matrix Multiply1/2
  Matrix Multiply1/1 -> Sum1/2
  Sum1/1 -> Sum/1
  In1/1 -> Sum1/1
  Matrix Multiply/1 -> Out1/1
  Sum/1 -> Matrix Multiply/2
  gyroCalBiases/1 -> Sum/2
  gyroCalMatrix/1 -> Matrix Multiply/1

== system ImuCalibrator3Pass/secondPass/printTime ==
  time : Inport
  Enable : EnablePort
  MATLAB Function : MATLAB Function  TreatAsAtomicUnit=on
  wires:
  time/1 -> MATLAB Function/1(u)

== system ImuCalibrator3Pass/secondPass/readImuData ==
  C++ S-function : S-Function  FunctionName=readImuData  Parameters=-1  SFunctionDeploymentMode=off  EnableBusSupport=off
  Constant : Constant  Value=0
  Constant1 : Constant
  Data Store Read : DataStoreRead  DataStoreName=SensorTypeIdentifier
  Data Store Write : DataStoreWrite  DataStoreName=cal_file_name
  Data Type Conversion : DataTypeConversion
  Data Type Conversion1 : DataTypeConversion  OutDataTypeStr=uint8
  Difference1 : simulink/Discrete/Difference  ICPrevInput=0.0  OutMin=[]  OutMax=[]  OutDataType=fixdt(1, 16)  OutScaling=2^-10  DoSatur=off
  Mux : Mux  Inputs=2
  SensorType : Selector  InputPortWidth=11  IndexOptions=Index vector (dialog)  Indices=2  OutputSizes=1
  Unit Delay : UnitDelay  SampleTime=-1
  Unit Delay1 : UnitDelay  SampleTime=-1
  avoid huge jump on first cycle : Switch  Criteria=u2 > Threshold  Threshold=0.5
  avoid sending garbage on the last row : Switch  Criteria=u2 > Threshold  Threshold=0.5
  gyros accels : Selector  InputPortWidth=11  IndexOptions=Index vector (dialog)  Indices=[5:10]  OutputSizes=1
  not initialized : simulink/Logic and Bit Operations/Compare To Constant  relop===  const=-1  OutDataTypeStr=boolean
  tstamp : Selector  InputPortWidth=11  IndexOptions=Index vector (dialog)  Indices=3  OutputSizes=1
  write SensorTypeIdentifier once : Subsystem  TreatAsAtomicUnit=on
  GyrosAccelsDt : Outport
  EOF : Outport  Port=2
  wires:
  tstamp/1 -> Difference1/1
  C++ S-function/1 -> gyros accels/1, SensorType/1, tstamp/1
  gyros accels/1 -> Mux/1
  SensorType/1 -> Data Type Conversion/1
  Data Store Read/1 -> not initialized/1
  not initialized/1 -> write SensorTypeIdentifier once/Enable
  Data Type Conversion/1 -> write SensorTypeIdentifier once/1(In1)
  Unit Delay/1 -> avoid sending garbage on the last row/1
  C++ S-function/2 -> avoid sending garbage on the last row/2, EOF/1
  avoid sending garbage on the last row/1 -> GyrosAccelsDt/1
  Mux/1 -> Unit Delay/1, avoid sending garbage on the last row/3
  Unit Delay1/1 -> avoid huge jump on first cycle/2
  Difference1/1 -> avoid huge jump on first cycle/1
  Constant/1 -> avoid huge jump on first cycle/3
  Constant1/1 -> Unit Delay1/1
  avoid huge jump on first cycle/1 -> Mux/2
  ? -> Data Type Conversion1/1
  Data Type Conversion1/1 -> Data Store Write/1

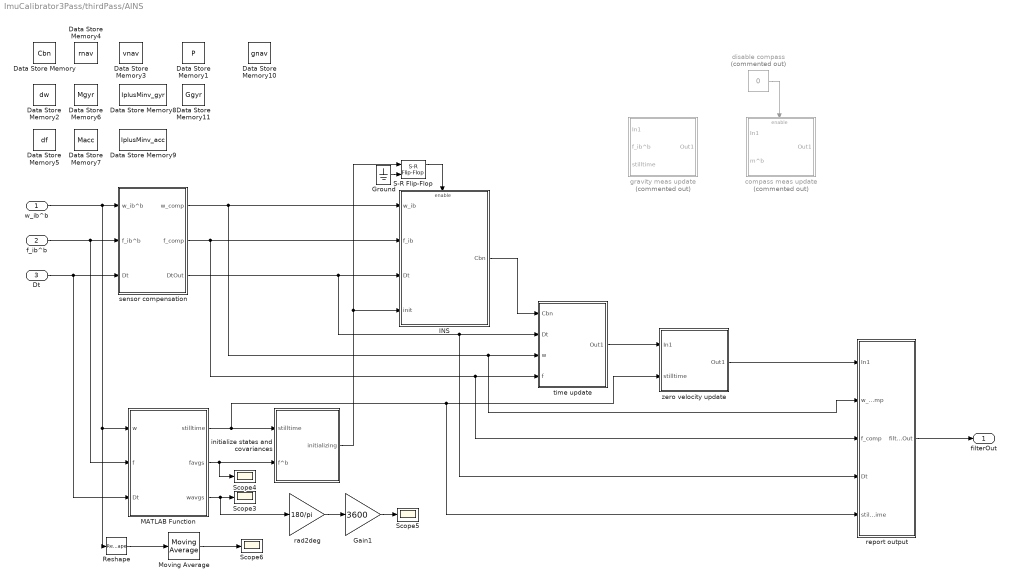
== system ImuCalibrator3Pass/thirdPass/AINS ==
  w_ib^b : Inport  Unit=rad/s
  f_ib^b : Inport  Port=2  Unit=m/s^2  PortDimensions=3
  Dt : Inport  Port=3  Unit=rad/s
  Data Store Memory : DataStoreMemory  DataStoreName=Cbn  ReadBeforeWriteMsg=warning  WriteAfterWriteMsg=warning  WriteAfterReadMsg=warning  InitialValue=eye(3)  VectorParams1D=off  ShowAdditionalParam=off
  Data Store Memory1 : DataStoreMemory  DataStoreName=P  ReadBeforeWriteMsg=warning  WriteAfterWriteMsg=warning  WriteAfterReadMsg=warning  InitialValue=eye(modelDef.numStates)*1e-12  ShowAdditionalParam=off
  Data Store Memory10 : DataStoreMemory  DataStoreName=gnav  ReadBeforeWriteMsg=warning  WriteAfterWriteMsg=warning  WriteAfterReadMsg=warning  InitialValue=[0;0; 9.8065]  VectorParams1D=off  ShowAdditionalParam=off
  Data Store Memory11 : DataStoreMemory  DataStoreName=Ggyr  ReadBeforeWriteMsg=warning  WriteAfterWriteMsg=warning  WriteAfterReadMsg=warning  InitialValue=zeros(3,3)  VectorParams1D=off  ShowAdditionalParam=off
  Data Store Memory2 : DataStoreMemory  DataStoreName=dw  ReadBeforeWriteMsg=warning  WriteAfterWriteMsg=warning  WriteAfterReadMsg=warning  InitialValue=[0;0;0]  VectorParams1D=off  ShowAdditionalParam=off
  Data Store Memory3 : DataStoreMemory  DataStoreName=vnav  ReadBeforeWriteMsg=warning  WriteAfterWriteMsg=warning  WriteAfterReadMsg=warning  InitialValue=[0;0;0]  VectorParams1D=off  ShowAdditionalParam=off
  Data Store Memory4 : DataStoreMemory  DataStoreName=rnav  ReadBeforeWriteMsg=warning  WriteAfterWriteMsg=warning  WriteAfterReadMsg=warning  InitialValue=[0;0;0]  VectorParams1D=off  ShowAdditionalParam=off
  Data Store Memory5 : DataStoreMemory  DataStoreName=df  ReadBeforeWriteMsg=warning  WriteAfterWriteMsg=warning  WriteAfterReadMsg=warning  InitialValue=[0;0;0]  VectorParams1D=off  ShowAdditionalParam=off
  Data Store Memory6 : DataStoreMemory  DataStoreName=Mgyr  ReadBeforeWriteMsg=warning  WriteAfterWriteMsg=warning  WriteAfterReadMsg=warning  InitialValue=zeros(3,3)  VectorParams1D=off  ShowAdditionalParam=off
  Data Store Memory7 : DataStoreMemory  DataStoreName=Macc  ReadBeforeWriteMsg=warning  WriteAfterWriteMsg=warning  WriteAfterReadMsg=warning  InitialValue=zeros(3,3)  VectorParams1D=off  ShowAdditionalParam=off
  Data Store Memory8 : DataStoreMemory  DataStoreName=IplusMinv_gyr  ReadBeforeWriteMsg=warning  WriteAfterWriteMsg=warning  WriteAfterReadMsg=warning  InitialValue=eye(3)  VectorParams1D=off  ShowAdditionalParam=off
  Data Store Memory9 : DataStoreMemory  DataStoreName=IplusMinv_acc  ReadBeforeWriteMsg=warning  WriteAfterWriteMsg=warning  WriteAfterReadMsg=warning  InitialValue=eye(3)  VectorParams1D=off  ShowAdditionalParam=off
  Gain1 : Gain  Gain=3600
  Ground : Ground
  INS : Subsystem  Priority=2
  MATLAB Function : MATLAB Function  TreatAsAtomicUnit=on
  Moving Average : dspstat3/Moving Average  Method=Sliding window  ForgettingFactorPort=off  SpecifyWindowLength=on  WindowLength=1000  ForgettingFactor=0.9  SimulateUsing=Code generation
  Reshape : Reshape  OutputDimensionality=Row vector (2-D)
  S-R Flip-Flop : simulink_extras/Flip Flops/S-R Flip-Flop  initial_condition=0
  Scope{3..6} (4 alike) : Scope
  compass meas update : Subsystem  Commented=on  TreatAsAtomicUnit=on
  disable compass : Constant  Commented=on  Value=0
  gravity meas update : Subsystem  Commented=on  TreatAsAtomicUnit=on
  initialize states and covariances : Subsystem  Priority=1  TreatAsAtomicUnit=on
  rad2deg : Gain  Gain=180/pi
  report output : Subsystem  Priority=10  TreatAsAtomicUnit=on
  sensor compensation : Subsystem
  time update : Subsystem  Priority=3  TreatAsAtomicUnit=on
  zero velocity update : Subsystem  Priority=4  TreatAsAtomicUnit=on
  filterOut : Outport
  wires:
  time update/1(Out1) -> zero velocity update/1(In1)
  disable compass/1 -> compass meas update/Enable
  MATLAB Function/1(stilltime) -> report output/5(stilltime), zero velocity update/2(stilltime), initialize states and covariances/1(stilltime)
  MATLAB Function/2(favgs) -> Scope4/1, initialize states and covariances/2(f^b)
  zero velocity update/1(Out1) -> report output/1(In1)
  sensor compensation/1(w_comp) -> report output/2(w_comp), time update/3(w), INS/1(w_ib)
  INS/1(Cbn) -> time update/1(Cbn)
  sensor compensation/3(DtOut) -> report output/4(Dt), time update/2(Dt), INS/3(Dt)
  sensor compensation/2(f_comp) -> INS/2(f_ib), report output/3(f_comp), time update/4(f)
  f_ib^b/1 -> MATLAB Function/2(f), sensor compensation/2(f_ib^b)
  w_ib^b/1 -> MATLAB Function/1(w), Reshape/1, sensor compensation/1(w_ib^b)
  Dt/1 -> MATLAB Function/3(Dt), sensor compensation/3(Dt)
  initialize states and covariances/1(initializing) -> INS/4(init), S-R Flip-Flop/1
  MATLAB Function/3(wavgs) -> rad2deg/1, Scope3/1
  rad2deg/1 -> Gain1/1
  Gain1/1 -> Scope5/1
  Moving Average/1 -> Scope6/1
  Reshape/1 -> Moving Average/1
  S-R Flip-Flop/1 -> INS/Enable
  report output/1(filterOut) -> filterOut/1
  Ground/1 -> S-R Flip-Flop/2

== system ImuCalibrator3Pass/thirdPass/apply accel calibration ==
  In1 : Inport
  accelCalBiases : Inport  Port=2
  accelCalMatrix : Inport  Port=3
  "Accel SFMA matrix, column-major1" : Constant  Value="[0.9973\t0.0126\t0.0025\t0.0004\t1.0177\t0.003\t0.0064\t0.0308\t1.0224]"  VectorParams1D=off
  Matrix Multiply : Product  Multiplication=Matrix(*)
  Sum : Sum  Inputs=|+-
  Out1 : Outport
  wires:
  In1/1 -> Sum/1
  Matrix Multiply/1 -> Out1/1
  Sum/1 -> Matrix Multiply/2
  accelCalBiases/1 -> Sum/2
  accelCalMatrix/1 -> Matrix Multiply/1

== system ImuCalibrator3Pass/thirdPass/apply gyro calibration ==
  gyroCalBiases : Inport
  gyroCalMatrix : Inport  Port=2
  gyroGsensMatrix : Inport  Port=3
  In1 : Inport  Port=4
  f : Inport  Port=5
  "Accel SFMA matrix, column-major1" : Constant  Value="[0.9973\t0.0126\t0.0025\t0.0004\t1.0177\t0.003\t0.0064\t0.0308\t1.0224]"  VectorParams1D=off
  Matrix Multiply : Product  Multiplication=Matrix(*)
  Matrix Multiply1 : Product  Multiplication=Matrix(*)
  Sum : Sum  Inputs=|+-
  Sum1 : Sum  Inputs=|+-
  Out1 : Outport
  wires:
  gyroCalMatrix/1 -> Matrix Multiply/1
  gyroCalBiases/1 -> Sum/2
  Sum/1 -> Matrix Multiply/2
  Matrix Multiply/1 -> Out1/1
  In1/1 -> Sum1/1
  Sum1/1 -> Sum/1
  Matrix Multiply1/1 -> Sum1/2
  f/1 -> Matrix Multiply1/2
  gyroGsensMatrix/1 -> Matrix Multiply1/1

== system ImuCalibrator3Pass/thirdPass/printTime ==
  time : Inport
  Enable : EnablePort
  MATLAB Function : MATLAB Function  TreatAsAtomicUnit=on
  wires:
  time/1 -> MATLAB Function/1(u)

== system ImuCalibrator3Pass/thirdPass/readImuData ==
  C++ S-function : S-Function  FunctionName=readImuData  Parameters=-1  SFunctionDeploymentMode=off  EnableBusSupport=off
  Constant : Constant  Value=0
  Constant1 : Constant
  Data Store Read : DataStoreRead  DataStoreName=SensorTypeIdentifier
  Data Store Write : DataStoreWrite  DataStoreName=cal_file_name
  Data Type Conversion : DataTypeConversion
  Data Type Conversion1 : DataTypeConversion  OutDataTypeStr=uint8
  Difference1 : simulink/Discrete/Difference  ICPrevInput=0.0  OutMin=[]  OutMax=[]  OutDataType=fixdt(1, 16)  OutScaling=2^-10  DoSatur=off
  Mux : Mux  Inputs=2
  SensorType : Selector  InputPortWidth=11  IndexOptions=Index vector (dialog)  Indices=2  OutputSizes=1
  Unit Delay : UnitDelay  SampleTime=-1
  Unit Delay1 : UnitDelay  SampleTime=-1
  avoid huge jump on first cycle : Switch  Criteria=u2 > Threshold  Threshold=0.5
  avoid sending garbage on the last row : Switch  Criteria=u2 > Threshold  Threshold=0.5
  gyros accels : Selector  InputPortWidth=11  IndexOptions=Index vector (dialog)  Indices=[5:10]  OutputSizes=1
  not initialized : simulink/Logic and Bit Operations/Compare To Constant  relop===  const=-1  OutDataTypeStr=boolean
  tstamp : Selector  InputPortWidth=11  IndexOptions=Index vector (dialog)  Indices=3  OutputSizes=1
  write SensorTypeIdentifier once : Subsystem  TreatAsAtomicUnit=on
  GyrosAccelsDt : Outport
  EOF : Outport  Port=2
  wires:
  tstamp/1 -> Difference1/1
  C++ S-function/1 -> gyros accels/1, SensorType/1, tstamp/1
  gyros accels/1 -> Mux/1
  SensorType/1 -> Data Type Conversion/1
  Data Store Read/1 -> not initialized/1
  not initialized/1 -> write SensorTypeIdentifier once/Enable
  Data Type Conversion/1 -> write SensorTypeIdentifier once/1(In1)
  Unit Delay/1 -> avoid sending garbage on the last row/1
  C++ S-function/2 -> avoid sending garbage on the last row/2, EOF/1
  avoid sending garbage on the last row/1 -> GyrosAccelsDt/1
  Mux/1 -> Unit Delay/1, avoid sending garbage on the last row/3
  Unit Delay1/1 -> avoid huge jump on first cycle/2
  Difference1/1 -> avoid huge jump on first cycle/1
  Constant/1 -> avoid huge jump on first cycle/3
  Constant1/1 -> Unit Delay1/1
  avoid huge jump on first cycle/1 -> Mux/2
  ? -> Data Type Conversion1/1
  Data Type Conversion1/1 -> Data Store Write/1

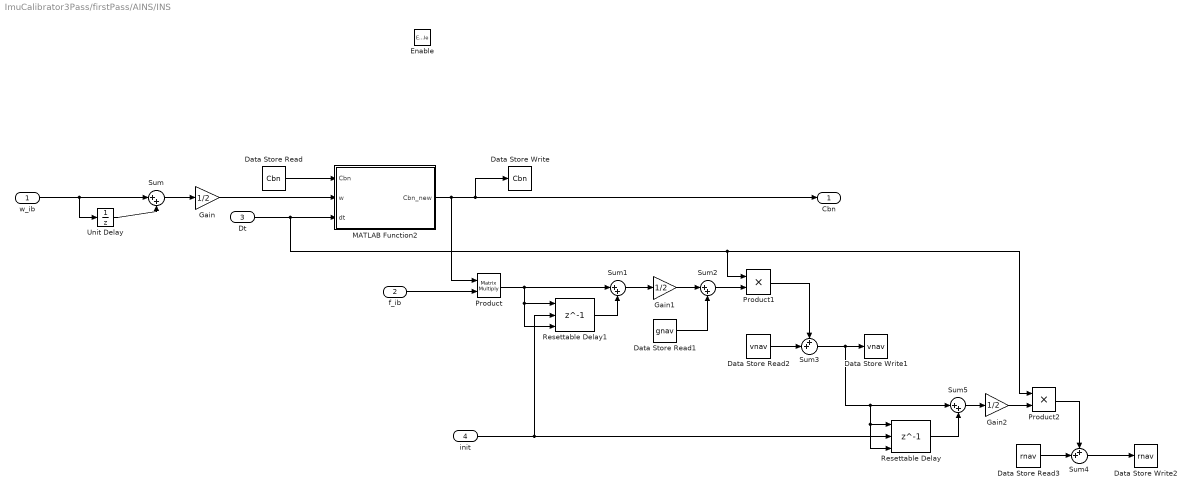
== system ImuCalibrator3Pass/firstPass/AINS/INS ==
  w_ib : Inport
  f_ib : Inport  Port=2
  Dt : Inport  Port=3
  init : Inport  Port=4
  Enable : EnablePort
  Data Store Read : DataStoreRead  DataStoreName=Cbn
  Data Store Read1 : DataStoreRead  DataStoreName=gnav
  Data Store Read2 : DataStoreRead  DataStoreName=vnav
  Data Store Read3 : DataStoreRead  DataStoreName=rnav
  Data Store Write : DataStoreWrite  DataStoreName=Cbn
  Data Store Write1 : DataStoreWrite  DataStoreName=vnav
  Data Store Write2 : DataStoreWrite  DataStoreName=rnav
  Gain : Gain  Gain=1/2
  Gain1 : Gain  Gain=1/2
  Gain2 : Gain  Gain=1/2
  MATLAB Function2 : MATLAB Function  TreatAsAtomicUnit=on
  Product : Product  Multiplication=Matrix(*)
  Product1 : Product
  Product2 : Product
  Resettable Delay : Delay  DelayLength=1  InitialConditionSource=Input port  ExternalReset=Level
      settings: InputPortMap=u0,r5,p4
  Resettable Delay1 : Delay  DelayLength=1  InitialConditionSource=Input port  ExternalReset=Level
      settings: InputPortMap=u0,r5,p4
  Sum{,1..2,5} (4 alike) : Sum  Inputs=|++
  Sum3 : Sum  Inputs=++|
  Sum4 : Sum  Inputs=++|
  Unit Delay : UnitDelay  SampleTime=-1
  Cbn : Outport
  wires:
  Dt/1 -> Product2/1, Product1/1, MATLAB Function2/3(dt)
  Data Store Read/1 -> MATLAB Function2/1(Cbn)
  w_ib/1 -> Unit Delay/1, Sum/1
  MATLAB Function2/1(Cbn_new) -> Product/1, Cbn/1, Data Store Write/1
  Unit Delay/1 -> Sum/2
  Sum/1 -> Gain/1
  Gain/1 -> MATLAB Function2/2(w)
  f_ib/1 -> Product/2
  Data Store Read1/1 -> Sum2/2
  Sum2/1 -> Product1/2
  Product/1 -> Resettable Delay1/3, Resettable Delay1/1, Sum1/1
  Sum1/1 -> Gain1/1
  Gain1/1 -> Sum2/1
  Data Store Read2/1 -> Sum3/2
  Product1/1 -> Sum3/1
  Data Store Read3/1 -> Sum4/2
  Sum4/1 -> Data Store Write2/1
  Sum5/1 -> Gain2/1
  Sum3/1 -> Resettable Delay/3, Resettable Delay/1, Sum5/1, Data Store Write1/1
  Gain2/1 -> Product2/2
  Resettable Delay/1 -> Sum5/2
  init/1 -> Resettable Delay1/2, Resettable Delay/2
  Resettable Delay1/1 -> Sum1/2
  Product2/1 -> Sum4/1

== system ImuCalibrator3Pass/firstPass/AINS/compass meas update ==
  note: this is just to enforce block execution order
  In1 : Inport
  m^b : Inport  Port=2
  Enable : EnablePort
  Data Store Read1 : DataStoreRead  DataStoreName=Cbn
  Data Store Read3 : DataStoreRead  DataStoreName=P
  Data Store Write : DataStoreWrite  DataStoreName=P
  Demux : Demux  Outputs=3
  Gain : Gain  Gain=-1
  H : Constant  Value=[ 0 0 1]  VectorParams1D=off
  MATLAB Function1 : MATLAB Function  TreatAsAtomicUnit=on
  MATLAB Function3 : MATLAB Function  TreatAsAtomicUnit=on
  Product : Product  Multiplication=Matrix(*)
  Product1 : Product  Multiplication=Matrix(*)
  R assumes 10 deg rms compass noise : Constant  Value=0.34^2
  Scope : Scope
  Scope1 : Scope
  Scope2 : Scope
  Trigonometric Function : Trigonometry  Operator=atan2
  update the Cbn with the errors : Subsystem
  Out1 : Outport
  wires:
  Product1/1 -> update the Cbn with the errors/1(phi  rotation errors), Scope/1  "phi  rotation errors"
  R assumes 10 deg rms compass noise/1 -> MATLAB Function1/3(R), MATLAB Function3/4(R)
  Data Store Read3/1 -> MATLAB Function1/1(P), MATLAB Function3/1(P)
  m^b/1 -> Product/2
  MATLAB Function3/1(Pplus) -> Data Store Write/1
  MATLAB Function1/2(K) -> Product1/1, MATLAB Function3/2(K), Scope2/1
  Trigonometric Function/1 -> Gain/1  "nu = 0 - psi"
  Product/1 -> Demux/1  "m^nhat"
  Data Store Read1/1 -> Product/1  "Cbn hat"
  In1/1 -> Out1/1
  Demux/2 -> Trigonometric Function/1
  Demux/1 -> Trigonometric Function/2
  H/1 -> MATLAB Function1/2(H), MATLAB Function3/3(H)
  Gain/1 -> Product1/2, Scope1/1
